simulink model "Controller4_PL"  (R2021b)
settings: Solver=VariableStepAuto  StartTime=0.0  StopTime=10.0  RelTol=1e-3
libraries: simulink_extras x3
settings Model: Creator=david  LastModifiedBy=david

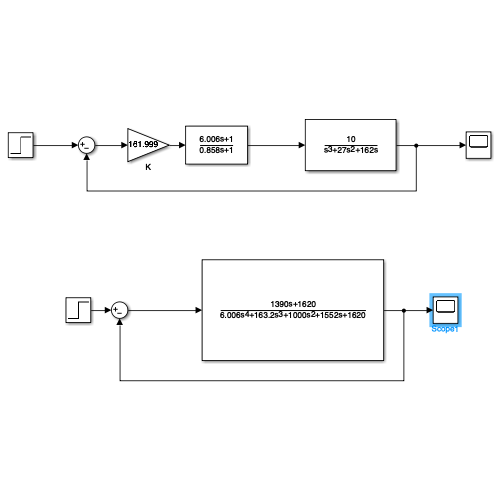
[thumbnail: Simulink's stored preview of the top-level diagram]
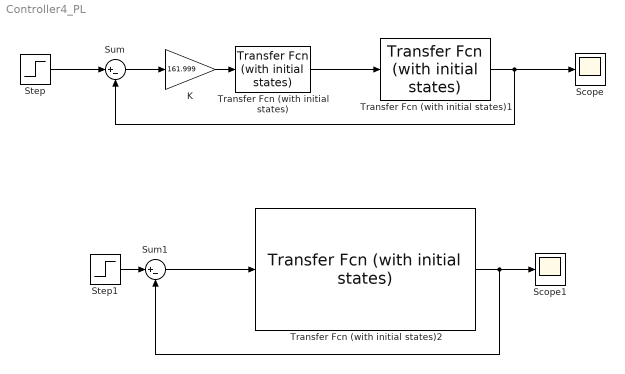
== system Controller4_PL ==
  K : Gain  Gain=161.999
  Scope : Scope
  Scope1 : Scope
  Step : Step  SampleTime=0
  Step1 : Step  SampleTime=0
  Sum : Sum  Inputs=|+-
  Sum1 : Sum  Inputs=|+-
  Transfer Fcn (with initial states) : simulink_extras/Additional Linear/Transfer Fcn (with initial states)  N=[6.006 1]  D=[.858 1]  X0=0
  Transfer Fcn (with initial states)1 : simulink_extras/Additional Linear/Transfer Fcn (with initial states)  N=[10]  D="[1  27 162 0]"  X0=0
  Transfer Fcn (with initial states)2 : simulink_extras/Additional Linear/Transfer Fcn (with initial states)  N=[1390 1620]  D=[6.006 163.2 1000 1552 1620]  X0=0
  wires:
  Transfer Fcn (with initial states)/1 -> Transfer Fcn (with initial states)1/1
  K/1 -> Transfer Fcn (with initial states)/1
  Transfer Fcn (with initial states)1/1 -> Scope/1, Sum/2
  Sum/1 -> K/1
  Step/1 -> Sum/1
  Sum1/1 -> Transfer Fcn (with initial states)2/1
  Transfer Fcn (with initial states)2/1 -> Scope1/1, Sum1/2
  Step1/1 -> Sum1/1
